simulink model "simulation_strecke_stoerung"  (Simulink 7.0)
settings: Solver=ode45  StartTime=0.0  StopTime=10.0  RelTol=1e-3
settings Model: Creator=Matze  LastModifiedBy=Matze

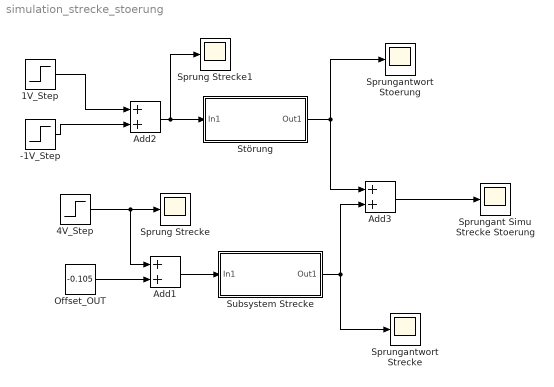
== system simulation_strecke_stoerung ==
  -1V_Step : Step  Time=6.9  After=-0.35  SampleTime=0
  1V_Step : Step  Time=4.5  After=0.35  SampleTime=0
  4V_Step : Step  After=4  SampleTime=0
  Add1 : Sum  OutDataType=sfix(16)  OutScaling=2^-10
  Add2 : Sum  OutDataType=sfix(16)  OutScaling=2^-10
  Add3 : Sum  OutDataType=sfix(16)  OutScaling=2^-10
  Offset_OUT : Constant  Value=-0.105  OutDataType=sfix(16)  OutScaling=2^0
  Sprung Strecke : Scope
      settings: TimeRange=10  YMin=0
  Sprung Strecke1 : Scope
      settings: TimeRange=10  YMin=0  SaveName=ScopeData2
  Sprungant Simu Strecke Stoerung : Scope
  Sprungantwort Stoerung : Scope
      settings: TimeRange=10  YMin=0  SaveName=ScopeData3
  Sprungantwort Strecke : Scope
      settings: TimeRange=10  YMin=0  SaveName=ScopeData4
  Störung : Subsystem
  Subsystem Strecke : Subsystem
  wires:
  4V_Step/1 -> Add1/1, Sprung Strecke/1
  Add1/1 -> Subsystem Strecke/1(In1)
  1V_Step/1 -> Add2/1
  -1V_Step/1 -> Add2/2
  Add2/1 -> Störung/1(In1), Sprung Strecke1/1
  Störung/1(Out1) -> Add3/1, Sprungantwort Stoerung/1
  Subsystem Strecke/1(Out1) -> Add3/2, Sprungantwort Strecke/1
  Add3/1 -> Sprungant Simu Strecke Stoerung/1
  Offset_OUT/1 -> Add1/2

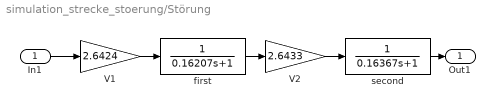
== system simulation_strecke_stoerung/Störung ==
  In1 : Inport  OutDataType=sfix(16)  OutScaling=2^0
  V1 : Gain  Gain=2.6424  ParameterDataType=sfix(16)  ParameterScaling=2^0  OutDataType=sfix(16)  OutScaling=2^0
  V2 : Gain  Gain=2.6433  ParameterDataType=sfix(16)  ParameterScaling=2^0  OutDataType=sfix(16)  OutScaling=2^0
  first : TransferFcn  Denominator=[0.16207 1]
  second : TransferFcn  Denominator=[0.16367 1]
  Out1 : Outport  OutDataType=sfix(16)  OutScaling=2^0
  wires:
  In1/1 -> V1/1
  V1/1 -> first/1
  first/1 -> V2/1
  second/1 -> Out1/1
  V2/1 -> second/1

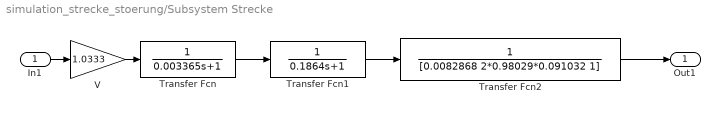
== system simulation_strecke_stoerung/Subsystem Strecke ==
  In1 : Inport  OutDataType=sfix(16)  OutScaling=2^0
  Transfer Fcn : TransferFcn  Denominator=[0.003365 1]
  Transfer Fcn1 : TransferFcn  Denominator=[0.1864 1]
  Transfer Fcn2 : TransferFcn  Denominator=[0.0082868 2*0.98029*0.091032 1]
  V : Gain  Gain=1.0333  ParameterDataType=sfix(16)  ParameterScaling=2^0  OutDataType=sfix(16)  OutScaling=2^0
  Out1 : Outport  OutDataType=sfix(16)  OutScaling=2^0
  wires:
  In1/1 -> V/1
  V/1 -> Transfer Fcn/1
  Transfer Fcn/1 -> Transfer Fcn1/1
  Transfer Fcn1/1 -> Transfer Fcn2/1
  Transfer Fcn2/1 -> Out1/1
